simulink model "p2"  (R2019a)
settings: Solver=VariableStepAuto  StartTime=0.0  StopTime=10.0  RelTol=1e-6
settings Model: Creator=jz73  LastModifiedBy=jz73

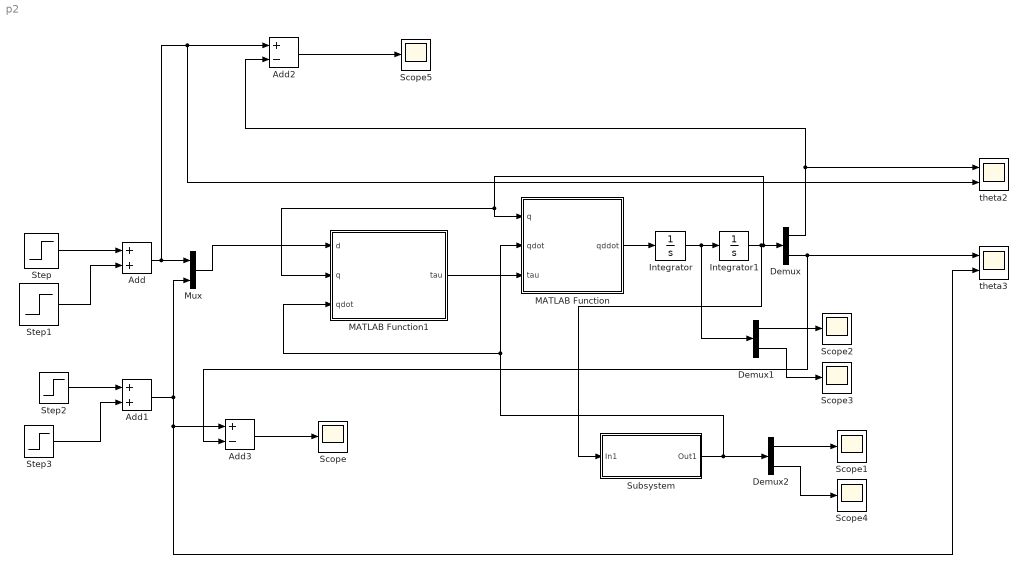
== system p2 ==
  Add : Sum
  Add1 : Sum
  Add2 : Sum  Inputs=+-
  Add3 : Sum  Inputs=+-
  Demux : Demux  Outputs=2
  Demux1 : Demux  Outputs=2
  Demux2 : Demux  Outputs=2
  Integrator : Integrator  InitialCondition=[0 0]
  Integrator1 : Integrator  InitialCondition=[0 0]
  MATLAB Function : MATLAB Function  TreatAsAtomicUnit=on
  MATLAB Function1 : MATLAB Function  TreatAsAtomicUnit=on
  Mux : Mux  Inputs=2
  Scope{,1..5} (6 alike) : Scope
  Step : Step  After=pi/6  SampleTime=0
  Step1 : Step  Time=2  After=-pi/6  SampleTime=0
  Step2 : Step  After=pi/6  SampleTime=0
  Step3 : Step  Time=2  After=-pi/6  SampleTime=0
  Subsystem : Subsystem
  theta2 : Scope  NumInputPorts=2
  theta3 : Scope  NumInputPorts=2
  wires:
  Integrator/1 -> Demux1/1, Integrator1/1
  Demux/1 -> Add2/2, theta2/1
  Demux/2 -> Add3/2, theta3/1
  Integrator1/1 -> Subsystem/1(In1), MATLAB Function/1(q), MATLAB Function1/2(q), Demux/1
  Demux1/1 -> Scope2/1
  Demux1/2 -> Scope3/1
  MATLAB Function/1(qddot) -> Integrator/1
  Subsystem/1(Out1) -> MATLAB Function/2(qdot), MATLAB Function1/3(qdot), Demux2/1
  Demux2/2 -> Scope4/1
  Demux2/1 -> Scope1/1
  Step/1 -> Add/1
  Step1/1 -> Add/2
  Step2/1 -> Add1/1
  Step3/1 -> Add1/2
  MATLAB Function1/1(tau) -> MATLAB Function/3(tau)
  Add1/1 -> Add3/1, theta3/2, Mux/2
  Add/1 -> theta2/2, Add2/1, Mux/1
  Mux/1 -> MATLAB Function1/1(d)
  Add2/1 -> Scope5/1
  Add3/1 -> Scope/1

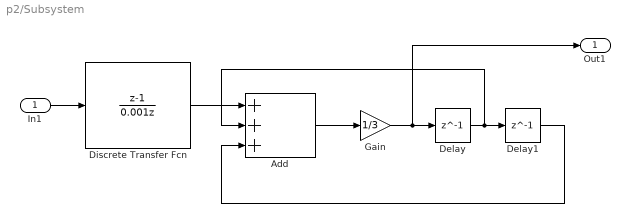
== system p2/Subsystem ==
  In1 : Inport
  Add : Sum  Inputs=+++
  Delay : Delay  DelayLength=1  InitialCondition=0  SampleTime=0.001
  Delay1 : Delay  DelayLength=1  InitialCondition=0  SampleTime=0.001
  Discrete Transfer Fcn : DiscreteTransferFcn  Numerator=[1 -1]  Denominator=[0.001 0]  SampleTime=0.001
  Gain : Gain  Gain=1/3
  Out1 : Outport
  wires:
  In1/1 -> Discrete Transfer Fcn/1
  Add/1 -> Gain/1
  Gain/1 -> Out1/1, Delay/1
  Delay/1 -> Add/2, Delay1/1
  Delay1/1 -> Add/3
  Discrete Transfer Fcn/1 -> Add/1

== matlab function p2/MATLAB Function1 ==
  data: d input; tau output; q input; qdot input
function tau = fcn(d, q,qdot)
    kp=80;
    kd=3;
    t=kp*(d-q)-kd*qdot;
tau = t;

== matlab function p2/MATLAB Function ==
  data: q input; qddot output; qdot input; tau input
function qddot = fcn(q,qdot,tau)
    p1=0.0300; 
    p2=0.0128; 
    p3=0.0076;
    p4=0.0753; 
    p5=0.0298;
    g=9.8;
    
    D=[p1 -p3*sin(q(2)-q(1));
     -p3*sin(q(2)-q(1)) p2];
    C=[0 -p3*cos(q(2)-q(1))*qdot(2);
        p3*cos(q(2)-q(1))*qdot(1) 0];
    G=[-p4*g*sin(q(1));-p5*g*cos(q(2))];
    u=inv(D)*(tau-C*qdot-G);
    
qddot = u;
